simulink model "untitled1"  (R2024b)
settings: Solver=VariableStepAuto  StartTime=0.0  StopTime=10  RelTol=1e-3
undefined symbols (not defined in the file): dspblkCoreblockFVToolHelper, G_z_001, G_z_01, G_z_1, gcbh
libraries: spsFourierLib x6, simulink x1
settings Model: Creator=SIGMA  LastModifiedBy=SIGMA

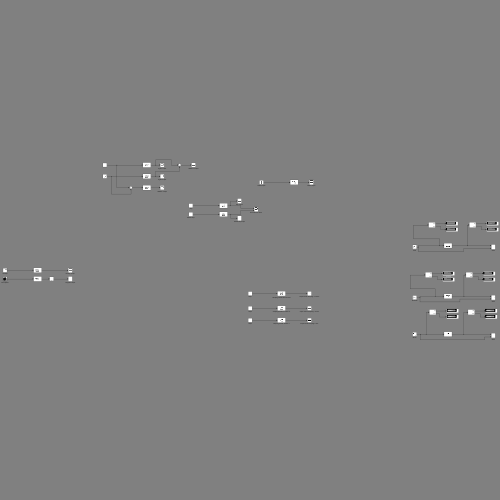
[thumbnail: Simulink's stored preview of the top-level diagram]
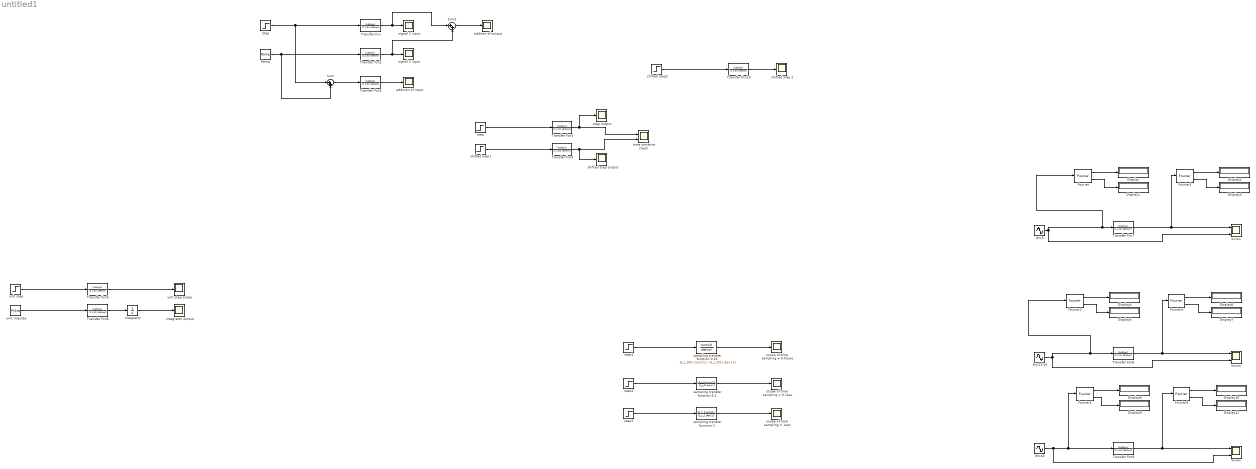
== system untitled1 ==
  " sampling transfer function 0.01" : DiscreteTransferFcn  LoadFcn=dspblkCoreblockFVToolHelper(gcbh,'load');  Numerator=G_z_001.num{1}  Denominator=G_z_001.den{1}
      settings: CopyFcn=dspblkCoreblockFVToolHelper(gcbh,'copy');  DeleteFcn=dspblkCoreblockFVToolHelper(gcbh,'close');  ModelCloseFcn=dspblkCoreblockFVToolHelper(gcbh,'close');  PreSaveFcn=dspblkCoreblockFVToolHelper(gcbh,'presave');  PostSaveFcn=dspblkCoreblockFVToolHelper(gcbh,'postsave');  CloseFcn=dspblkCoreblockFVToolHelper(gcbh,'close');
  " sampling transfer function 0.1" : DiscreteTransferFcn  LoadFcn=dspblkCoreblockFVToolHelper(gcbh,'load');  Numerator=G_z_01.num{1}  Denominator=G_z_01.den{1}
      settings: CopyFcn=dspblkCoreblockFVToolHelper(gcbh,'copy');  DeleteFcn=dspblkCoreblockFVToolHelper(gcbh,'close');  ModelCloseFcn=dspblkCoreblockFVToolHelper(gcbh,'close');  PreSaveFcn=dspblkCoreblockFVToolHelper(gcbh,'presave');  PostSaveFcn=dspblkCoreblockFVToolHelper(gcbh,'postsave');  CloseFcn=dspblkCoreblockFVToolHelper(gcbh,'close');
  " sampling transfer function 1" : DiscreteTransferFcn  LoadFcn=dspblkCoreblockFVToolHelper(gcbh,'load');  Numerator=G_z_1.num{1}  Denominator=G_z_1.den{1}
      settings: CopyFcn=dspblkCoreblockFVToolHelper(gcbh,'copy');  DeleteFcn=dspblkCoreblockFVToolHelper(gcbh,'close');  ModelCloseFcn=dspblkCoreblockFVToolHelper(gcbh,'close');  PreSaveFcn=dspblkCoreblockFVToolHelper(gcbh,'presave');  PostSaveFcn=dspblkCoreblockFVToolHelper(gcbh,'postsave');  CloseFcn=dspblkCoreblockFVToolHelper(gcbh,'close');
  " step" : Step  Time=0  After=10  SampleTime=0
  " step1" : Step  Time=0  SampleTime=0.01
  " step2" : Step  Time=0  SampleTime=0.1
  " step3" : Step  Time=0  SampleTime=1
  " unit step" : Step  Time=0  SampleTime=0
  " w<wn" : Scope  NumInputPorts=2
  " w=wn" : Scope  NumInputPorts=2
  " w>wn" : Scope  NumInputPorts=2
  Display{,1..11} (12 alike) : Display
  Fourier : spsFourierLib/Fourier  Freq=5/(2*pi)  n=1  InInit=[0, 0]  Ts=0
  Fourier1 : spsFourierLib/Fourier  Freq=5/(2*pi)  n=1  InInit=[0, 0]  Ts=0
  Fourier2 : spsFourierLib/Fourier  Freq=22.56/(2*pi)  n=1  InInit=[0, 0]  Ts=0
  Fourier3 : spsFourierLib/Fourier  Freq=22.56/(2*pi)  n=1  InInit=[0, 0]  Ts=0
  Fourier4 : spsFourierLib/Fourier  Freq=40/(2*pi)  n=1  InInit=[0, 0]  Ts=0
  Fourier5 : spsFourierLib/Fourier  Freq=40/(2*pi)  n=1  InInit=[0, 0]  Ts=0
  Integrator : Integrator
  Ramp : simulink/Sources/Ramp  slope=5  start=1  InitialOutput=0
  Step : Step  After=10  SampleTime=0
  Sum : Sum  Inputs=|++
  Sum1 : Sum  Inputs=|++
  Transfer Fcn{,1..10} (11 alike) : TransferFcn  Numerator=[1600/pi]  Denominator=[1 1.32 1600/pi]
  W=22.56 : Sin  Frequency=22.56  SampleTime=0  VectorParams1D=off
  W=40 : Sin  Frequency=40  SampleTime=0  VectorParams1D=off
  W=5 : Sin  Frequency=5  SampleTime=0  VectorParams1D=off
  addition of input : Scope
  additon of output : Scope
  integrator output : Scope
  scope of time sampling = 0.01sec : Scope
  scope of time sampling = 0.1sec : Scope
  scope of time sampling = 1sec : Scope
  shifted step 2 : Scope
  shifted step output : Scope
  shifted step1 : Step  Time=2  After=10  SampleTime=0
  shifted step2 : Step  Time=3  After=10  SampleTime=0
  signal 1 input : Scope
  signal 2 input : Scope
  step output : Scope
  time variance check : Scope  NumInputPorts=2
  unit impulse : DiscretePulseGenerator  PulseType=Time based  Amplitude=50  Period=20  PulseWidth=0.1
  "unit step scope " : Scope
  wires:
  Step/1 -> Sum/1, Transfer Fcn/1
  Ramp/1 -> Transfer Fcn1/1, Sum/2
  Sum/1 -> Transfer Fcn2/1
  Transfer Fcn2/1 -> addition of input/1
  Transfer Fcn/1 -> Sum1/1, signal 1 input/1
  Transfer Fcn1/1 -> Sum1/2, signal 2 input/1
  Sum1/1 -> additon of output/1
  " step"/1 -> Transfer Fcn3/1
  Transfer Fcn3/1 -> time variance check/1, step output/1
  shifted step1/1 -> Transfer Fcn4/1
  Transfer Fcn4/1 -> shifted step output/1, time variance check/2
  " unit step"/1 -> Transfer Fcn5/1
  Transfer Fcn5/1 -> "unit step scope "/1
  unit impulse/1 -> Transfer Fcn6/1
  Transfer Fcn6/1 -> Integrator/1
  W=5/1 -> Fourier/1, Transfer Fcn7/1, " w<wn"/2
  shifted step2/1 -> Transfer Fcn10/1
  Transfer Fcn10/1 -> shifted step 2/1
  Integrator/1 -> integrator output/1
  " step1"/1 -> " sampling transfer function 0.01"/1
  " sampling transfer function 0.01"/1 -> scope of time sampling = 0.01sec/1
  " sampling transfer function 0.1"/1 -> scope of time sampling = 0.1sec/1
  " step2"/1 -> " sampling transfer function 0.1"/1
  " sampling transfer function 1"/1 -> scope of time sampling = 1sec/1
  " step3"/1 -> " sampling transfer function 1"/1
  Fourier/1 -> Display/1
  Fourier/2 -> Display1/1
  Fourier1/2 -> Display3/1
  Transfer Fcn7/1 -> Fourier1/1, " w<wn"/1
  Fourier1/1 -> Display2/1
  Fourier2/2 -> Display5/1
  Transfer Fcn8/1 -> Fourier3/1, " w=wn"/1
  Fourier3/2 -> Display7/1
  W=22.56/1 -> " w=wn"/2, Fourier2/1, Transfer Fcn8/1
  Fourier3/1 -> Display6/1
  Fourier2/1 -> Display4/1
  Fourier5/1 -> Display10/1
  Fourier4/1 -> Display8/1
  Fourier5/2 -> Display11/1
  Fourier4/2 -> Display9/1
  W=40/1 -> " w>wn"/2, Transfer Fcn9/1, Fourier4/1
  Transfer Fcn9/1 -> Fourier5/1, " w>wn"/1
